simulink model "Pacemaker_A1"  (R2022b)
settings: Solver=FixedStepAuto  StartTime=0.0  StopTime=10.0  FixedStep=1e-3  RelTol=1e-3  EnableMultiTasking=on
undefined symbols (not defined in the file): D0, D1, D10, D11, D12, D13, D2, D3, D4, D5, D6, D7, D8, D9, PTA0, PTA1, PTA2, PTB23, PTB9, PTC16, PTC17, PTC2, PTC3, PTC4, PTD0, PTD1, PTD2, PTD3
libraries: frdmk64flib x17
settings Model: ExtModeTrigDuration=5  Creator=27161  LastModifiedBy=27161
settings SolverCC: AlgebraicLoopSolver=TrustRegion
settings OptimizationCC: EnhancedBackFolding=on  PassReuseOutputArgsAs=Individual arguments  ZeroExternalMemoryAtStartup=off  ZeroInternalMemoryAtStartup=off  MaxStackSize=64  OptimizeBlockOrder=speed  DifferentSizesBufferReuse=on  OptimizationCustomize=off  EfficientTunableParamExpr=on
settings DebuggingCC: ParameterTunabilityLossMsg=error  UnconnectedInputMsg=warning  UnconnectedOutputMsg=warning  UnconnectedLineMsg=warning  SFMachineParentedDataDiag=warning
settings HardwareCC: ProdBitPerPointer=32  ProdBitPerSizeT=32  ProdBitPerPtrDiffT=32  ProdLargestAtomicInteger=Long  ProdLargestAtomicFloat=Double  ProdWordSize=32  ProdHWDeviceType=ARM Compatible->ARM Cortex
settings ModelReferenceCC: EnableRefExpFcnMdlSchedulingChecks=on
settings SFSimCC: MATLABDynamicMemAlloc=off
settings RTWCC: Description=Embedded Coder  SystemTargetFile=ert.tlc  HardwareBoard=NXP FRDM-K64F  TLCOptions="-aInlineSetEventsForThisBaseRateFcn=TLC_FALSE -aSuppressMultiTaskScheduler=TLC_FALSE  -aRateBasedStepFcn=0"  TemplateMakefile=ert_default_tmf  Toolchain=GNU Tools for ARM Embedded Processors
settings CodeAppCC: ForceParamTrailComments=on  IgnoreCustomStorageClasses=off  OperatorAnnotations=on  SimulinkDataObjDesc=on  SFDataObjDesc=on  InsertBlockDesc=on

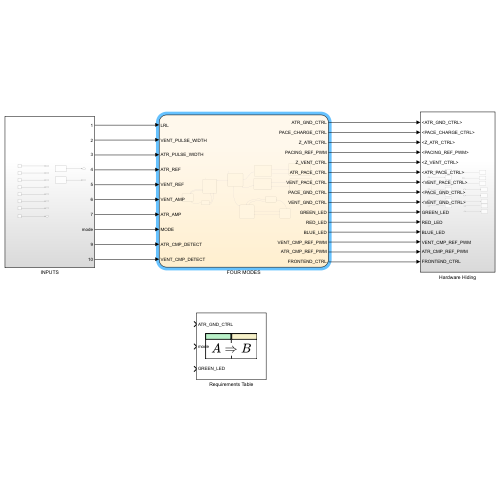
[thumbnail: Simulink's stored preview of the top-level diagram]
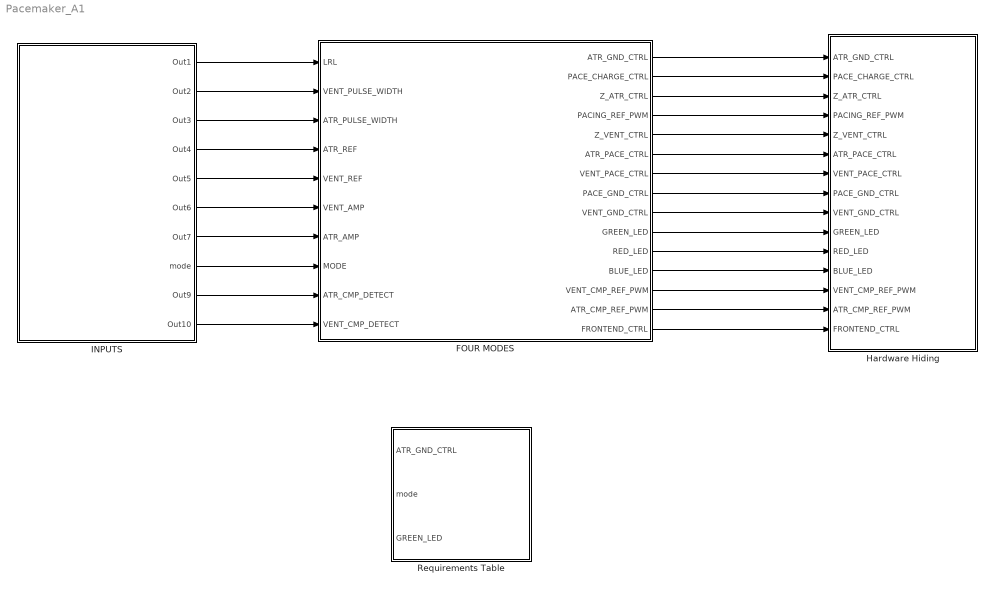
== system Pacemaker_A1 ==
  FOUR MODES : Stateflow chart  TreatAsAtomicUnit=on
      settings: PortSchema="{\"entries\":[{\"content\":{\"sides\":[{\"content\":{\"connectorIds\":[\"In1\",\"In3\",\"In2\",\"In7\",\"In4\",\"In6\",\"In8\",\"In9\",\"In10\",\"In5\"]},\"type\":\"ConnectorPlacement.EquallySpacedRectSide\",\"uuid\":\"6661be6b-aedb-4592-878a-fd9116f5820d\"},{\"content\":{\"connectorIds\":[\"Out9\",\"Out1\",\"Out2\",\"Out3\",\"Out4\",\"Out5\",\"Out6\",\"Out8\",\"Out7\",\"Out12\",\"Out13\",\"Out11\",\"Out14\",\"Out15\",\"Out10\"],\"side\":\"RIGHT\"},\"type\":\"ConnectorPlacement.EquallySpacedRectSide\",\"uuid\":\"f16586c3-0c99-4971-ba5f-75b93d25059c\"},{\"content\":{\"connectorIds\":[],\"side\":\"TOP\"},\"type\":\"ConnectorPlacement.EquallySpacedRectSide\",\"uuid\":\"27cb1bd0-c170-4ecc-a4df-3797e7aecef3\"}]},\"type\":\"ConnectorPlacement.EquallySpacedConnector\",\"uuid\":\"03557791-41f4-4916-8cde-1fcab0cf663d\"}],\"packageUris\":[\"http://schema.mathworks.com/mf0/Connector/R2020b\"],\"version\":\"1.0\"}"
  Hardware Hiding : Subsystem
  INPUTS : Subsystem
  Requirements Table : Requirements Table  TreatAsAtomicUnit=on
  wires:
  FOUR MODES/2(Z_ATR_CTRL) -> Hardware Hiding/3(Z_ATR_CTRL)
  FOUR MODES/9(ATR_GND_CTRL) -> Hardware Hiding/1(ATR_GND_CTRL)
  FOUR MODES/1(PACE_CHARGE_CTRL) -> Hardware Hiding/2(PACE_CHARGE_CTRL)
  FOUR MODES/3(PACING_REF_PWM) -> Hardware Hiding/4(PACING_REF_PWM)
  FOUR MODES/4(Z_VENT_CTRL) -> Hardware Hiding/5(Z_VENT_CTRL)
  FOUR MODES/5(ATR_PACE_CTRL) -> Hardware Hiding/6(ATR_PACE_CTRL)
  FOUR MODES/6(VENT_PACE_CTRL) -> Hardware Hiding/7(VENT_PACE_CTRL)
  FOUR MODES/7(VENT_GND_CTRL) -> Hardware Hiding/9(VENT_GND_CTRL)
  FOUR MODES/8(PACE_GND_CTRL) -> Hardware Hiding/8(PACE_GND_CTRL)
  INPUTS/1(Out1) -> FOUR MODES/1(LRL)
  INPUTS/2(Out2) -> FOUR MODES/3(VENT_PULSE_WIDTH)
  INPUTS/3(Out3) -> FOUR MODES/2(ATR_PULSE_WIDTH)
  INPUTS/4(Out4) -> FOUR MODES/7(ATR_REF)
  INPUTS/5(Out5) -> FOUR MODES/4(VENT_REF)
  INPUTS/6(Out6) -> FOUR MODES/6(VENT_AMP)
  INPUTS/8(mode) -> FOUR MODES/9(MODE)
  INPUTS/7(Out7) -> FOUR MODES/8(ATR_AMP)
  INPUTS/10(Out10) -> FOUR MODES/5(VENT_CMP_DETECT)
  FOUR MODES/12(GREEN_LED) -> Hardware Hiding/10(GREEN_LED)
  INPUTS/9(Out9) -> FOUR MODES/10(ATR_CMP_DETECT)
  FOUR MODES/15(ATR_CMP_REF_PWM) -> Hardware Hiding/14(ATR_CMP_REF_PWM)
  FOUR MODES/14(VENT_CMP_REF_PWM) -> Hardware Hiding/13(VENT_CMP_REF_PWM)
  FOUR MODES/13(RED_LED) -> Hardware Hiding/11(RED_LED)
  FOUR MODES/11(BLUE_LED) -> Hardware Hiding/12(BLUE_LED)
  FOUR MODES/10(FRONTEND_CTRL) -> Hardware Hiding/15(FRONTEND_CTRL)

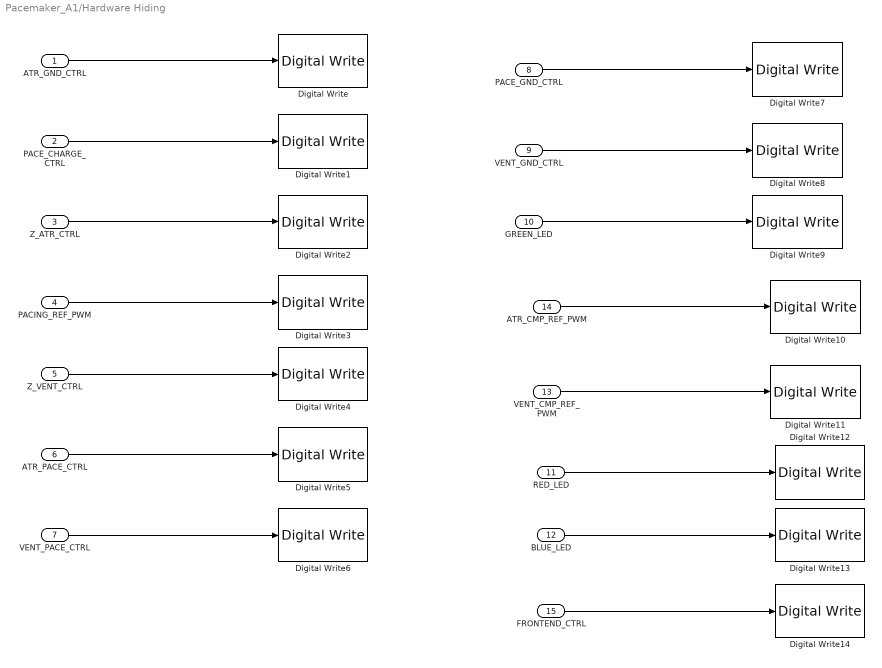
== system Pacemaker_A1/Hardware Hiding ==
  ATR_GND_CTRL : Inport
  PACE_CHARGE_CTRL : Inport  Port=2
  Z_ATR_CTRL : Inport  Port=3
  PACING_REF_PWM : Inport  Port=4
  Z_VENT_CTRL : Inport  Port=5
  ATR_PACE_CTRL : Inport  Port=6
  VENT_PACE_CTRL : Inport  Port=7
  PACE_GND_CTRL : Inport  Port=8
  VENT_GND_CTRL : Inport  Port=9
  GREEN_LED : Inport  Port=10
  RED_LED : Inport  Port=11
  BLUE_LED : Inport  Port=12
  VENT_CMP_REF_PWM : Inport  Port=13
  ATR_CMP_REF_PWM : Inport  Port=14
  FRONTEND_CTRL : Inport  Port=15
  Digital Write : frdmk64flib/Digital Write  Whichpin=PTD2 (D11)
  Digital Write1 : frdmk64flib/Digital Write  Whichpin=PTB9 (D2)
  Digital Write10 : frdmk64flib/Digital Write  Whichpin=PTA1 (D3)
  Digital Write11 : frdmk64flib/Digital Write  Whichpin=PTC2 (D6)
  Digital Write12 : frdmk64flib/Digital Write  Whichpin=RED_LED
  Digital Write13 : frdmk64flib/Digital Write  Whichpin=BLUE_LED
  Digital Write14 : frdmk64flib/Digital Write  Whichpin=PTD1 (D13)
  Digital Write2 : frdmk64flib/Digital Write  Whichpin=PTB23 (D4)
  Digital Write3 : frdmk64flib/Digital Write  Whichpin=PTA2 (D5)
  Digital Write4 : frdmk64flib/Digital Write  Whichpin=PTC3 (D7)
  Digital Write5 : frdmk64flib/Digital Write  Whichpin=PTA0 (D8)
  Digital Write6 : frdmk64flib/Digital Write  Whichpin=PTC4 (D9)
  Digital Write7 : frdmk64flib/Digital Write  Whichpin=PTD0 (D10)
  Digital Write8 : frdmk64flib/Digital Write  Whichpin=PTD3 (D12)
  Digital Write9 : frdmk64flib/Digital Write  Whichpin=GREEN_LED
  wires:
  ATR_GND_CTRL/1 -> Digital Write/1
  PACE_CHARGE_CTRL/1 -> Digital Write1/1
  Z_ATR_CTRL/1 -> Digital Write2/1
  PACING_REF_PWM/1 -> Digital Write3/1
  Z_VENT_CTRL/1 -> Digital Write4/1
  ATR_PACE_CTRL/1 -> Digital Write5/1
  VENT_PACE_CTRL/1 -> Digital Write6/1
  PACE_GND_CTRL/1 -> Digital Write7/1
  VENT_GND_CTRL/1 -> Digital Write8/1
  GREEN_LED/1 -> Digital Write9/1
  ATR_CMP_REF_PWM/1 -> Digital Write10/1
  VENT_CMP_REF_PWM/1 -> Digital Write11/1
  RED_LED/1 -> Digital Write12/1
  BLUE_LED/1 -> Digital Write13/1
  FRONTEND_CTRL/1 -> Digital Write14/1

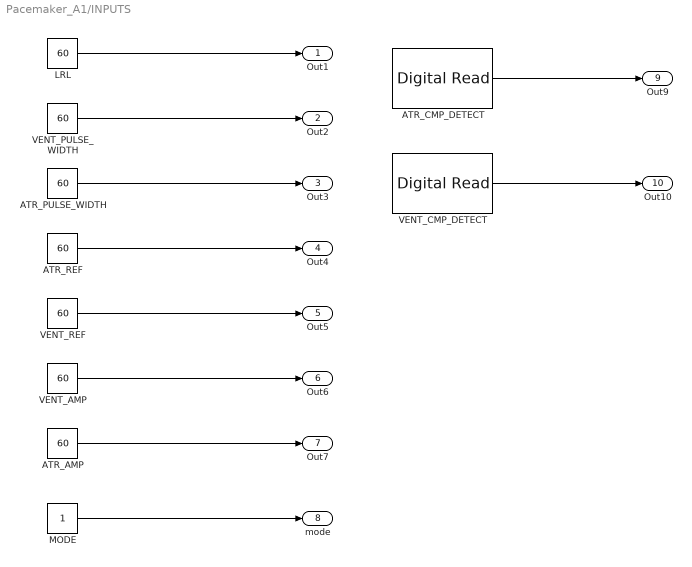
== system Pacemaker_A1/INPUTS ==
  ATR_AMP : Constant  Value=60
  ATR_CMP_DETECT : frdmk64flib/Digital Read  Whichpin=PTC16 (D0)  SampleTime=-1
  ATR_PULSE_WIDTH : Constant  Value=60
  ATR_REF : Constant  Value=60
  LRL : Constant  Value=60
  MODE : Constant
  VENT_AMP : Constant  Value=60
  VENT_CMP_DETECT : frdmk64flib/Digital Read  Whichpin=PTC17 (D1)  SampleTime=-1
  VENT_PULSE_WIDTH : Constant  Value=60
  VENT_REF : Constant  Value=60
  Out1 : Outport
  Out2 : Outport  Port=2
  Out3 : Outport  Port=3
  Out4 : Outport  Port=4
  Out5 : Outport  Port=5
  Out6 : Outport  Port=6
  Out7 : Outport  Port=7
  mode : Outport  Port=8
  Out9 : Outport  Port=9
  Out10 : Outport  Port=10
  wires:
  LRL/1 -> Out1/1
  VENT_PULSE_WIDTH/1 -> Out2/1
  ATR_PULSE_WIDTH/1 -> Out3/1
  ATR_REF/1 -> Out4/1
  VENT_REF/1 -> Out5/1
  VENT_AMP/1 -> Out6/1
  ATR_AMP/1 -> Out7/1
  MODE/1 -> mode/1
  ATR_CMP_DETECT/1 -> Out9/1
  VENT_CMP_DETECT/1 -> Out10/1

== stateflow chart Pacemaker_A1/Requirements Table ==
  (default) -> (junction 1073741860)
  (junction 1073741860) -> (junction 1073741861) : {
      | % SF_REQ_REV_07
      | }
  (junction 1073741861) -> (junction 1073741863) : {
      | % HEADER_ASSIGNMENTS
      |
      | }
  (junction 1073741863) -> (junction 1073741865) : {
      | % START_A_4
      | }
  (junction 1073741865) -> (junction 1073741867) : {
      | }
  (junction 1073741867) -> (junction 1073741869)
  (junction 1073741869) -> (junction 1073741871) : {
      | }
  (junction 1073741871) -> (junction 1073741873) : {
      | % END_A_4
      | }
  (junction 1073741873) -> (junction 1073741934) : {
      | % START_R_1
      | }
  (junction 1073741934) -> (junction 1073741936) : {
      | }
  (junction 1073741936) -> (junction 1073741938)
  (junction 1073741938) -> (junction 1073741940) [order 1] : [(((mode) == (1)))]
  (junction 1073741938) -> (junction 1073741956) [order 2]
  (junction 1073741940) -> (junction 1073741942) : {
      |
      |
      | }
  (junction 1073741942) -> (junction 1073741944) : {
      | }
  (junction 1073741944) -> (junction 1073741946) : {
      | % START_R_7
      | }
  (junction 1073741946) -> (junction 1073741948) : {
      | }
  (junction 1073741948) -> (junction 1073741950) : {
      |
      |
      | }
  (junction 1073741950) -> (junction 1073741952) : {
      | }
  (junction 1073741952) -> (junction 1073741973) : {
      | % END_R_7
      | }
  (junction 1073741973) -> (junction 1073741956)
  (junction 1073741956) -> (junction 1073741958)
  (junction 1073741958) -> (junction 1073741960) : {
      | % END_R_1
      | }
  (junction 1073741960) -> (junction 1073742022) : {
      | % START_R_10
      | }
  (junction 1073742022) -> (junction 1073742024) : {
      | }
  (junction 1073742024) -> (junction 1073742026)
  (junction 1073742026) -> (junction 1073742028) [order 1] : [(((mode) == (2)))]
  (junction 1073742026) -> (junction 1073742034) [order 2]
  (junction 1073742028) -> (junction 1073742030) : {
      |
      |
      | }
  (junction 1073742030) -> (junction 1073742032) : {
      | }
  (junction 1073742032) -> (junction 1073742034)
  (junction 1073742034) -> (junction 1073742036)
  (junction 1073742036) -> (junction 1073742038) : {
      | % END_R_10
      | }
  (junction 1073742038) -> (junction 1073742076) : {
      | % START_R_13
      | }
  (junction 1073742076) -> (junction 1073742078) : {
      | }
  (junction 1073742078) -> (junction 1073742080)
  (junction 1073742080) -> (junction 1073742082) [order 1] : [(((mode) == (3)))]
  (junction 1073742080) -> (junction 1073742098) [order 2]
  (junction 1073742082) -> (junction 1073742084) : {
      | reqtable_postcondition((((PACE_CHARGE_CTRL) == (true))), 'R:3');
      |
      |
      | }
  (junction 1073742084) -> (junction 1073742086) : {
      | }
  (junction 1073742086) -> (junction 1073742107) : {
      | % START_R_19
      | }
  (junction 1073742107) -> (junction 1073742109) : {
      | }
  (junction 1073742109) -> (junction 1073742111)
  (junction 1073742111) -> (junction 1073742113) [order 1] : [(((VENT_CMP_DETECT) == (false)))]
  (junction 1073742111) -> (junction 1073742119) [order 2]
  (junction 1073742113) -> (junction 1073742115) : {
      | reqtable_postcondition((((FRONTED_CTRL) == (true))) && (((PACE_CHARGE_CTRL) == (false))), 'R:3.1');
      |
      |
      | }
  (junction 1073742115) -> (junction 1073742117) : {
      | }
  (junction 1073742117) -> (junction 1073742119)
  (junction 1073742119) -> (junction 1073742121)
  (junction 1073742121) -> (junction 1073742123) : {
      | % END_R_19
      | }
  (junction 1073742123) -> (junction 1073742140) : {
      | % START_R_22
      | }
  (junction 1073742140) -> (junction 1073742142) : {
      | }
  (junction 1073742142) -> (junction 1073742144)
  (junction 1073742144) -> (junction 1073742146) [order 1] : [(((VENT_CMP_DETECT) == (true)))]
  (junction 1073742144) -> (junction 1073742152) [order 2]
  (junction 1073742146) -> (junction 1073742148) : {
      | reqtable_postcondition((((RED_LED) == (true))) && (((FRONTED_CTRL) == (false))) && (((PACE_CHARGE_CTRL) == (false))), 'R:3.2');
      |
      |
      | }
  (junction 1073742148) -> (junction 1073742150) : {
      | }
  (junction 1073742150) -> (junction 1073742152)
  (junction 1073742152) -> (junction 1073742154)
  (junction 1073742154) -> (junction 1073742156) : {
      | % END_R_22
      | }
  (junction 1073742156) -> (junction 1073742098)
  (junction 1073742098) -> (junction 1073742100)
  (junction 1073742100) -> (junction 1073742102) : {
      | % END_R_13
      | }
  (junction 1073742102) -> (junction 1073742055) : {
      | % START_R_16
      | }
  (junction 1073742055) -> (junction 1073742057) : {
      | }
  (junction 1073742057) -> (junction 1073742059)
  (junction 1073742059) -> (junction 1073742061) [order 1] : [(((mode) == (4)))]
  (junction 1073742059) -> (junction 1073742067) [order 2]
  (junction 1073742061) -> (junction 1073742063) : {
      |
      |
      | }
  (junction 1073742063) -> (junction 1073742065) : {
      | }
  (junction 1073742065) -> (junction 1073742067)
  (junction 1073742067) -> (junction 1073742069)
  (junction 1073742069) -> (junction 1073742071) : {
      | % END_R_16
      | }
  data: ATR_GND_CTRL input; mode input; GREEN_LED input

== stateflow chart Pacemaker_A1/FOUR MODES ==
  state AOO_PACING
    %Discharge C22 and charge block/C21
    PACE_CHARGE_CTRL = false;
    PACE_GND_CTRL = true;
    ATR_PACE_CTRL = true;
    ATR_GND_CTRL = false;
    Z_ATR_CTRL = false;
    Z_VENT_CTRL = false;
    VENT_GND_CTRL = false;
    VENT_PACE_CTRL = false;
    GREEN_LED =0; %check state
  state AOO_INITIAL
    entry:
    %Charge C22, discharge block/C21
    ATR_PACE_CTRL = false;
    ATR_GND_CTRL = true;
    VENT_GND_CTRL = false;
    VENT_PACE_CTRL = false;
    PACE_CHARGE_CTRL = true;
    PACE_GND_CTRL = true;
    Z_ATR_CTRL = false;
    Z_VENT_CTRL = false;
    PACING_REF_PWM = ATR_AMP*20
    GREEN_LED = 1; %check state
  state MainState
    entry:
    ATR_PACE_CTRL = false;
    ATR_GND_CTRL = false;
    VENT_GND_CTRL = false;
    VENT_PACE_CTRL = false;
    PACE_CHARGE_CTRL = false;
    PACE_GND_CTRL = false;
    Z_ATR_CTRL = false;
    Z_VENT_CTRL = false;
    FRONTEND_CTRL = false;
    %verify it is at initial state
    BLUE_LED = 1
  state VOO_INITIAL
    entry:
    %Charge C22, discharge block
    ATR_PACE_CTRL = false;
    ATR_GND_CTRL = false;
    VENT_GND_CTRL = true;
    VENT_PACE_CTRL = false;
    PACE_CHARGE_CTRL = true;
    PACE_GND_CTRL = true;
    Z_ATR_CTRL = false;
    Z_VENT_CTRL = false;
    PACING_REF_PWM = VENT_AMP*20
    RED_LED = 1; %check state
  state VOO_PACING
    %Discharge C22 and charge block/C21
    PACE_CHARGE_CTRL = false;
    PACE_GND_CTRL = true;
    ATR_PACE_CTRL = false;
    ATR_GND_CTRL = false;
    Z_ATR_CTRL = false;
    Z_VENT_CTRL = false;
    VENT_GND_CTRL = false;
    VENT_PACE_CTRL = true;
    BLUE_LED =0;%check state
  note: In the initial state of AAI, we have
      | sensor on to detact if the input voltage is higher
      | than our set threshlod.
      |
      | We also charge C22 for possible pacing
      | state happen when not detection of natural
      | pulse, and discharge C21 to end the pacing state.
      |
      | LED light is off at initial state.
  state AAI_INITIAL
    entry:
    FRONTEND_CTRL= true;
    ATR_PACE_CTRL = false;
    VENT_PACE_CTRL = false;
    PACING_REF_PWM = ATR_AMP*20;
    PACE_CHARGE_CTRL = true;
    Z_ATR_CTRL = false;
    Z_VENT_CTRL = false;
    PACE_GND_CTRL = true;
    VENT_GND_CTRL = false;
    ATR_GND_CTRL = true;
    GREEN_LED = 1;
    ATR_CMP_REF_PWM = 70;
  note: When no detect natural pulse, pace the atrium
      | with connecting C22 to C11. Then wait for 1 cycle.
  state AAI_PACING
    entry:
    PACE_CHARGE_CTRL = false;
    PACE_GND_CTRL = true;
    ATR_PACE_CTRL = true;
    ATR_GND_CTRL = false;
    Z_ATR_CTRL = false;
    Z_VENT_CTRL = false;
    VENT_GND_CTRL = false;
    VENT_PACE_CTRL = false;
    RED_LED = 1;
  note: In the Refractory state, sensor turn off.
      | A signal of this happen will have red LED turn on.
      | After a refractory period, go back to initial state.
  state VVI_REF
    entry:
    FRONTEND_CTRL = false;
    PACE_CHARGE_CTRL = false;
    BLUE_LED = 1;
  state AAI_REF
    entry:
    FRONTEND_CTRL = false;
    PACE_CHARGE_CTRL = false;
    BLUE_LED = 1;
  state VVI_INITIAL
    entry:
    FRONTEND_CTRL= true;%sensor on
    %charge C22, discharge C21
    Z_ATR_CTRL = false;
    Z_VENT_CTRL = false;
    PACE_GND_CTRL = true;
    VENT_GND_CTRL = true;
    ATR_GND_CTRL = false;
    ATR_PACE_CTRL = false;
    VENT_PACE_CTRL = false;
    PACE_CHARGE_CTRL = true;
    PACING_REF_PWM = VENT_AMP*20;
    RED_LED = 1;
    VENT_CMP_REF_PWM = 70;
  note: In the Refractory state, sensor turn off.
      | A signal of this happen will have red LED turn on.
      | After a refractory period, go back to initial state.
  note: In the initial state of VVI, we turn the
      | sensor on to detect if the input voltage is higher
      | than our set threshlod.
      |
      | We also charge C22 for possible pacing
      | state happen when not detection of natural
      | pulse, and discharge C21 to end the pacing state.
      |
      | LED light is off at initial state.
  state VVI_PACING
    entry:
    %same as VOO pacing
    %discharge C22 and charge C21
    PACE_CHARGE_CTRL = false;
    PACE_GND_CTRL = true;
    ATR_PACE_CTRL = false;
    ATR_GND_CTRL = false;
    Z_ATR_CTRL = false;
    Z_VENT_CTRL = false;
    VENT_GND_CTRL = false;
    VENT_PACE_CTRL = true;
    GREEN_LED = 1;
  AOO_INITIAL -> AOO_PACING : [after(60000/LRL - ATR_PULSE_WIDTH,msec)]
  (default) -> MainState [order 1]
  MainState -> AOO_INITIAL [order 1] : [mode == 1]
  AOO_PACING -> AOO_INITIAL : [after(ATR_PULSE_WIDTH,msec)]
  (default) -> AAI_INITIAL [order 2]
  MainState -> AAI_INITIAL [order 4] : [mode == 4]
  VOO_INITIAL -> VOO_PACING : [after(60000/LRL - VENT_PULSE_WIDTH,msec)]
  MainState -> VOO_INITIAL [order 2] : [mode == 2]
  VOO_PACING -> VOO_INITIAL : [after(VENT_PULSE_WIDTH,msec)]
  MainState -> VVI_INITIAL [order 3] : [mode == 3]
  AAI_INITIAL -> AAI_PACING [order 1] : [ATR_CMP_DETECT == false && after(60000/LRL - ATR_PULSE_WIDTH,msec)]
  AAI_PACING -> AAI_INITIAL [order 2] : [after(ATR_PULSE_WIDTH,msec)]
  AAI_INITIAL -> AAI_REF [order 2] : [ATR_CMP_DETECT == true]
  AAI_REF -> AAI_INITIAL : [after(ATR_REF, msec)]
  VVI_REF -> VVI_INITIAL : [after(VENT_REF, msec)]
  VVI_PACING -> VVI_REF [order 1] : [VENT_CMP_DETECT == true]
  VVI_INITIAL -> VVI_REF [order 2] : [VENT_CMP_DETECT == true]
  AAI_PACING -> AAI_REF [order 1] : [ATR_CMP_DETECT == true]
  VVI_INITIAL -> VVI_PACING [order 1] : [VENT_CMP_DETECT ==false && after(60000/LRL - VENT_PULSE_WIDTH,msec)]
  VVI_PACING -> VVI_INITIAL [order 2] : [after(VENT_PULSE_WIDTH,msec)]
  data: PACE_CHARGE_CTRL output; Z_ATR_CTRL output; PACING_REF_PWM output; Z_VENT_CTRL output; ATR_PACE_CTRL output; VENT_PACE_CTRL output; VENT_GND_CTRL output; PACE_GND_CTRL output; ATR_GND_CTRL output; LRL input; ATR_PULSE_WIDTH input; VENT_PULSE_WIDTH input; FRONTEND_CTRL output; BLUE_LED output; GREEN_LED output; VENT_REF input; VENT_CMP_DETECT input; VENT_AMP input; ATR_REF input; RED_LED output; ATR_AMP input; MODE input; VENT_CMP_REF_PWM output; ATR_CMP_DETECT input; ATR_CMP_REF_PWM output
